simulink library "Valve_ThermoTset_fn"  (Simulink 8.2)
settings: Solver=ode45  StartTime=0.0  StopTime=10.0  RelTol=1e-3
libraries: carnot x2
settings Model: Creator=lena.frank  LastModifiedBy=drhf

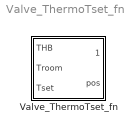
== system Valve_ThermoTset_fn ==
  Valve_ThermoTset_fn : Subsystem  mask(thermostatic valve with Kv function){p=3, op=0.5, bl=0.1, ts=30, dia=0.02, kv=0.6, kvs=0.8}
      mask prompts: p "proportional Range [K]"; op "operating point [0..1] (valve position at set temperature)"; bl "play hysteresis [K]"; ts "first-order hold ts [s]"; dia "diameter [m]"; kv "kv value"; kvs "kvs value"
      mask help:
      | Thermostatic valve for a radiator.
      | set temperature and slope
      | valve position = -slope * (T(sensor) - Toffset)
      mask Help: web(fullfile(path_carnot('help'),'Valve_Thermostatic.html'),'-helpbrowser')
      mask Display:
      | plot(-30,-10,130,110,[20,80,80,20,20],[60,30,60,30,60],[50,50],[45,70],[60,40],[96,96],[50,50],[75,96])
      | % port_label('input',1,'THB')
      | % port_label('input',2,'Troom')
      | % port_label('input',3,'Tset')
      | % port_label('output',1,'THB')

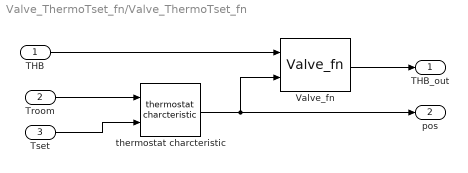
== system Valve_ThermoTset_fn/Valve_ThermoTset_fn ==
  THB : Inport
  Troom : Inport  Port=2
  Tset : Inport  Port=3
  Valve_fn : carnot/Hydraulics/Valve_fn  kv=kv  kvs=kvs  op=op
  thermostat charcteristic : carnot/Hydraulics/Valve_ThermoTset/thermostat charcteristic
  THB_out : Outport  InitialOutput=0
  pos : Outport  Port=2  InitialOutput=0
  wires:
  Valve_fn/1 -> THB_out/1
  Troom/1 -> thermostat charcteristic/1
  Tset/1 -> thermostat charcteristic/2
  THB/1 -> Valve_fn/1
  thermostat charcteristic/1 -> pos/1, Valve_fn/2
